simulink model "MaIA_SDCI_Temperature_Control"  (R2025b)
settings: Solver=VariableStepAuto  StartTime=0.0  StopTime=1800  RelTol=1e-3
PreLoadFcn:
  | %% MaIA_SDCI - Model Preload Callback
  | % Keep this callback intentionally minimal.
  | % All portable initialization logic lives in startup_project.m.
  | 
  | modelFile = get_param(bdroot, 'FileName');
  | 
  | if isempty(modelFile)
  |     error('MaIA_SDCI:ModelFileNotFound', ...
  |         'Unable to determine the current model file location.');
  | end
  | 
  | projectRoot = fileparts(modelFile);
  | addpath(projectRoot, '-begin');
  | rehash path;
  | startup_project(projectRoot);
InitFcn:
  | %% ============================================================
  | %  SIMULATION LAUNCH SOURCE
  | %  ============================================================
  | 
  | % false -> Run initiated directly from Simulink
  | % true  -> Run initiated from the MaIA_SDCI GUI
  | %
  | % Do not overwrite this variable if it already exists because
  | % the GUI sets it to true immediately before starting a run.
  | 
  | if ~evalin( ...
  |         'base', ...
  |         'exist(''MaIA_SDCI_RUN_FROM_GUI'',''var'')')
  | 
  |     assignin( ...
  |         'base', ...
  |         'MaIA_SDCI_RUN_FROM_GUI', ...
  |         false);
  | 
  | end
StartFcn:
  | %% MaIA_SDCI - Simulation Start Callback
  | 
  | runFromGUI = false;
  | 
  | %% Check simulation origin
  | 
  | if evalin( ...
  |         'base', ...
  |         'exist(''MaIA_SDCI_RUN_FROM_GUI'',''var'')')
  | 
  |     flagValue = evalin( ...
  |         'base', ...
  |         'MaIA_SDCI_RUN_FROM_GUI');
  | 
  |     if islogical(flagValue) || isnumeric(flagValue)
  |         runFromGUI = logical(flagValue);
  |     end
  | 
  | end
  | 
  | %% Open or focus the control application
  | 
  | launch_app;
  | 
  | %% Manual Run from Simulink
  | 
  | if ~runFromGUI
  | 
  |     drawnow;
  | 
  |     set_param( ...
  |         bdroot, ...
  |         'SimulationCommand', ...
  |         'stop');
  | 
  | end
values from neighbouring files (symbols this model uses):
  CFG = project_config()    [startup_project.m]
  ENV = environment_parameters()    [startup_project.m]
  MODEL = model_parameters()    [startup_project.m]
  SENSOR = sensor_parameters()    [startup_project.m]
libraries: fl_lib x58, nesl_utility x38, simulink x2
(part 2 of 2)

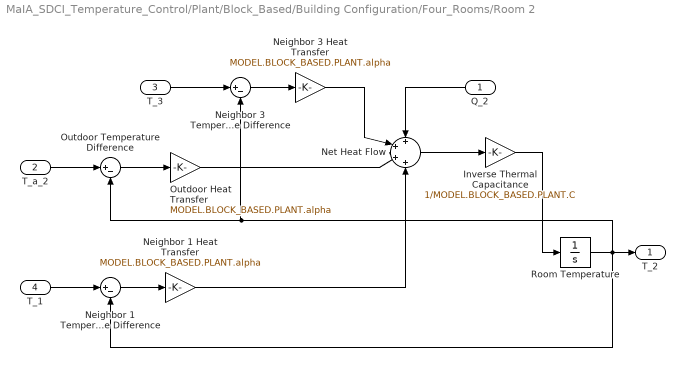
== system MaIA_SDCI_Temperature_Control/Plant/Block_Based/Building Configuration/Four_Rooms/Room 2 ==
  Q_2 : Inport
  T_a_2 : Inport  Port=2
  T_3 : Inport  Port=3
  T_1 : Inport  Port=4
  Inverse Thermal Capacitance : Gain  Gain=1/MODEL.BLOCK_BASED.PLANT.C
  Neighbor 1 Heat Transfer : Gain  Gain=MODEL.BLOCK_BASED.PLANT.alpha
  Neighbor 1 Temperature Difference : Sum  Inputs=|+-
  Neighbor 3 Heat Transfer : Gain  Gain=MODEL.BLOCK_BASED.PLANT.alpha
  Neighbor 3 Temperature Difference : Sum  Inputs=|+-
  Net Heat Flow : Sum  Inputs=++++
  Outdoor Heat Transfer : Gain  Gain=MODEL.BLOCK_BASED.PLANT.alpha
  Outdoor Temperature Difference : Sum  Inputs=|+-
  Room Temperature : Integrator  InitialCondition=MODEL.BLOCK_BASED.PLANT.initialTemperature(2)
  T_2 : Outport
  wires:
  Room Temperature/1 -> Neighbor 3 Temperature Difference/2, Outdoor Temperature Difference/2, T_2/1, Neighbor 1 Temperature Difference/2
  T_a_2/1 -> Outdoor Temperature Difference/1
  Outdoor Temperature Difference/1 -> Outdoor Heat Transfer/1
  T_1/1 -> Neighbor 1 Temperature Difference/1
  Neighbor 1 Temperature Difference/1 -> Neighbor 1 Heat Transfer/1
  T_3/1 -> Neighbor 3 Temperature Difference/1
  Neighbor 3 Temperature Difference/1 -> Neighbor 3 Heat Transfer/1
  Neighbor 3 Heat Transfer/1 -> Net Heat Flow/2
  Q_2/1 -> Net Heat Flow/1
  Neighbor 1 Heat Transfer/1 -> Net Heat Flow/4
  Outdoor Heat Transfer/1 -> Net Heat Flow/3
  Net Heat Flow/1 -> Inverse Thermal Capacitance/1
  Inverse Thermal Capacitance/1 -> Room Temperature/1

== system MaIA_SDCI_Temperature_Control/Plant/Block_Based/Building Configuration/Four_Rooms/Room 3 ==
  Q_3 : Inport
  T_a_3 : Inport  Port=2
  T_4 : Inport  Port=3
  T_2 : Inport  Port=4
  Inverse Thermal Capacitance : Gain  Gain=1/MODEL.BLOCK_BASED.PLANT.C
  Neighbor 2 Heat Transfer : Gain  Gain=MODEL.BLOCK_BASED.PLANT.alpha
  Neighbor 2 Temperature Difference : Sum  Inputs=|+-
  Neighbor 4 Heat Transfer : Gain  Gain=MODEL.BLOCK_BASED.PLANT.alpha
  Neighbor 4 Temperature Difference : Sum  Inputs=|+-
  Net Heat Flow : Sum  Inputs=++++
  Outdoor Heat Transfer : Gain  Gain=MODEL.BLOCK_BASED.PLANT.alpha
  Outdoor Temperature Difference : Sum  Inputs=|+-
  Room Temperature : Integrator  InitialCondition=MODEL.BLOCK_BASED.PLANT.initialTemperature(3)
  T_3 : Outport
  wires:
  Room Temperature/1 -> Neighbor 4 Temperature Difference/2, Outdoor Temperature Difference/2, T_3/1, Neighbor 2 Temperature Difference/2
  T_a_3/1 -> Outdoor Temperature Difference/1
  Outdoor Temperature Difference/1 -> Outdoor Heat Transfer/1
  T_2/1 -> Neighbor 2 Temperature Difference/1
  Neighbor 2 Temperature Difference/1 -> Neighbor 2 Heat Transfer/1
  T_4/1 -> Neighbor 4 Temperature Difference/1
  Neighbor 4 Temperature Difference/1 -> Neighbor 4 Heat Transfer/1
  Neighbor 4 Heat Transfer/1 -> Net Heat Flow/2
  Q_3/1 -> Net Heat Flow/1
  Neighbor 2 Heat Transfer/1 -> Net Heat Flow/4
  Outdoor Heat Transfer/1 -> Net Heat Flow/3
  Net Heat Flow/1 -> Inverse Thermal Capacitance/1
  Inverse Thermal Capacitance/1 -> Room Temperature/1

== system MaIA_SDCI_Temperature_Control/Plant/Block_Based/Building Configuration/Four_Rooms/Room 4 ==
  Q_4 : Inport
  T_a_4 : Inport  Port=2
  T_3 : Inport  Port=3
  Inverse Thermal Capacitance : Gain  Gain=1/MODEL.BLOCK_BASED.PLANT.C
  Neighbor 3 Heat Transfer : Gain  Gain=MODEL.BLOCK_BASED.PLANT.alpha
  Neighbor 3 Temperature Difference : Sum  Inputs=|+-
  Net Heat Flow : Sum  Inputs=|+++
  Outdoor Heat Transfer : Gain  Gain=MODEL.BLOCK_BASED.PLANT.alpha
  Outdoor Temperature Difference : Sum  Inputs=|+-
  Room Temperature : Integrator  InitialCondition=MODEL.BLOCK_BASED.PLANT.initialTemperature(4)
  T_4 : Outport
  wires:
  T_a_4/1 -> Outdoor Temperature Difference/1
  Room Temperature/1 -> Neighbor 3 Temperature Difference/2, T_4/1, Outdoor Temperature Difference/2
  Outdoor Temperature Difference/1 -> Outdoor Heat Transfer/1
  T_3/1 -> Neighbor 3 Temperature Difference/1
  Neighbor 3 Temperature Difference/1 -> Neighbor 3 Heat Transfer/1
  Outdoor Heat Transfer/1 -> Net Heat Flow/2
  Neighbor 3 Heat Transfer/1 -> Net Heat Flow/3
  Q_4/1 -> Net Heat Flow/1
  Net Heat Flow/1 -> Inverse Thermal Capacitance/1
  Inverse Thermal Capacitance/1 -> Room Temperature/1

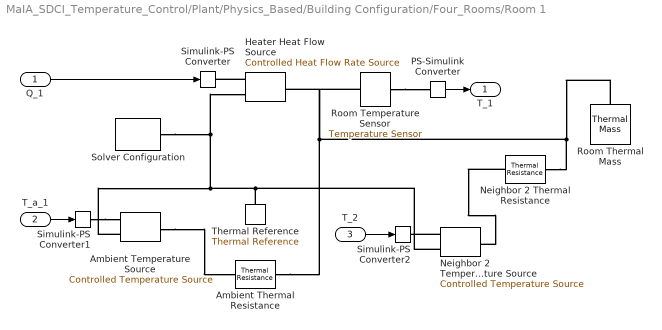
== system MaIA_SDCI_Temperature_Control/Plant/Physics_Based/Building Configuration/Four_Rooms/Room 1 ==
  Q_1 : Inport
  T_a_1 : Inport  Port=2
  T_2 : Inport  Port=3
  " Thermal Reference" : fl_lib/Thermal/Thermal Elements/Thermal Reference
  Ambient Temperature Source : fl_lib/Thermal/Thermal Sources/Controlled Temperature Source
  Ambient Thermal Resistance : fl_lib/Thermal/Thermal Elements/Thermal Resistance  resistance=1/MODEL.SIMSCAPE.PLANT.alpha K/W  T_specify=off  T_priority=None  T=0 K  T_nominal_specify=off  T_nominal_value=1  T_nominal_unit=K  Q_specify=off  Q_priority=None  Q=0 W  Q_nominal_specify=off  Q_nominal_value=1  Q_nominal_unit=W
  "Heater Heat Flow Source " : fl_lib/Thermal/Thermal Sources/Controlled Heat Flow Rate Source
  Neighbor 2 Temperature Source : fl_lib/Thermal/Thermal Sources/Controlled Temperature Source
  Neighbor 2 Thermal Resistance : fl_lib/Thermal/Thermal Elements/Thermal Resistance  resistance=1/MODEL.SIMSCAPE.PLANT.alpha K/W  T_specify=off  T_priority=None  T=0 K  T_nominal_specify=off  T_nominal_value=1  T_nominal_unit=K  Q_specify=off  Q_priority=None  Q=0 W  Q_nominal_specify=off  Q_nominal_value=1  Q_nominal_unit=W
  PS-Simulink Converter : nesl_utility/PS-Simulink Converter  PhysicalDomain=network_engine_domain  SubClassName=ps_output  LeftPortType=input  RightPortType=output  PseudoPeriodic=off  Frequencies=[]  VectorFormat=inherit  Unit=degC  AffineConversion=on
  Room Temperature Sensor : fl_lib/Thermal/Thermal Sensors/Temperature Sensor  temperature_measure=foundation.enum.MeasurementReference.absolute
      settings: InternalSimscapePortConfiguration="{\"Bottom\":[],\"Left\":[{\"id\":\"A\",\"label\":\"A\",\"type\":\"foundation.thermal.thermal\"}],\"Right\":[{\"id\":\"T\",\"label\":\"T\",\"type\":\"output\"}],\"Top\":[]}"
  Room Thermal Mass : fl_lib/Thermal/Thermal Elements/Thermal Mass  mass_type=foundation.enum.constant_variable.constant  mass=1 kg  sp_heat=MODEL.SIMSCAPE.PLANT.C J/(K*kg)  mass_min=1e-6 kg  num_ports=foundation.enum.numPorts2.one  m_specify=off  m_priority=High  m=1 kg  m_nominal_specify=off  m_nominal_value=1  m_nominal_unit=kg  T_specify=on  T_priority=High  T=MODEL.SIMSCAPE.PLANT.initialTemperature(1) degC  T_nominal_specify=off  T_nominal_value=1  T_nominal_unit=K  Q_specify=off  Q_priority=None  Q=0 W  Q_nominal_specify=off  Q_nominal_value=1  Q_nominal_unit=W
  Simulink-PS Converter : nesl_utility/Simulink-PS Converter  PhysicalDomain=network_engine_domain  SubClassName=ps_input  LeftPortType=input  RightPortType=output  PseudoPeriodic=off  Frequencies=[]  NoiseDistribution=none  NoiseParameters=[]  Unit=W  AffineConversion=off  FilteringAndDerivatives=provide  SimscapeFilterOrder=1  InputFilterTimeConstant=0.001  UdotUserProvided=0
  Simulink-PS Converter1 : nesl_utility/Simulink-PS Converter  PhysicalDomain=network_engine_domain  SubClassName=ps_input  LeftPortType=input  RightPortType=output  PseudoPeriodic=off  Frequencies=[]  NoiseDistribution=none  NoiseParameters=[]  Unit=degC  AffineConversion=on  FilteringAndDerivatives=provide  SimscapeFilterOrder=1  InputFilterTimeConstant=0.001  UdotUserProvided=0
  Simulink-PS Converter2 : nesl_utility/Simulink-PS Converter  PhysicalDomain=network_engine_domain  SubClassName=ps_input  LeftPortType=input  RightPortType=output  PseudoPeriodic=off  Frequencies=[]  NoiseDistribution=none  NoiseParameters=[]  Unit=degC  AffineConversion=on  FilteringAndDerivatives=provide  SimscapeFilterOrder=1  InputFilterTimeConstant=0.001  UdotUserProvided=0
  "Solver Configuration " : nesl_utility/Solver Configuration  PhysicalDomain=network_engine_domain  SubClassName=solver  LeftPortType=input  RightPortType=generic  Tones=[]  Harmonics=[]  SimulateNoise=off  Profile=off  UseLocalSampling=off  EnableSwitchedLinearOptims=on  FrequencyDomain=off  UseCCode=off  RelTol=0.001  AbsTol=0.001  MinStep=1e-09  ToWorkspace=off  RevertToSquareIcSolve=off  NumHomotopyIterations=100  PhasorMode=off  PhasorModeNumHarmonics=1  ConsistencySolver=NEWTON_XTOL_AFTER_FTOL  IndexReductionMethod=DerivativeReplacement  DoDC=off  ResidualTolerance=1e-09  ConsistencyTolSource=GLOBAL  ConsistencyAbsTol=0.001  ConsistencyRelTol=0.001  ConsistencyTolFactor=0.001  UseLocalSolver=off  LocalSolverChoice=NE_BACKWARD_EULER_ADVANCER  ResolveIndetEquations=on  FunctionEvalNumThread=1  LocalSolverSampleTime=0.001  DoFixedCost=off  MaxNonlinIter=3  MaxModeIter=2  ComputeImpulses=off  ImpulseIterations=2  LinearAlgebra=auto  LinearAlgebraNumThread=0  EquationFormulation=NE_TIME_EF  DelaysMemoryBudget=1024  AutomaticFiltering=on  FilteringTimeConstant=0.001  PartitionStorageMethod=AS_NEEDED  PartitionMemoryBudget=1024  PartitionMethod=ROBUST  MultibodyUseLocalSolver=off  MultibodyLocalSolverChoice=ODE1  MultibodyLocalSolverSampleTime=0.001
  T_1 : Outport
  wires:
  Q_1/1 -> Simulink-PS Converter/1
  PS-Simulink Converter/1 -> T_1/1
  T_a_1/1 -> Simulink-PS Converter1/1
  T_2/1 -> Simulink-PS Converter2/1
  connections:
  "Heater Heat Flow Source "/RConn1 -- Simulink-PS Converter/RConn1
  Room Thermal Mass/LConn1 -- Room Temperature Sensor/LConn1 -- "Heater Heat Flow Source "/LConn1 -- Ambient Thermal Resistance/RConn1 -- Neighbor 2 Thermal Resistance/RConn1
  Room Temperature Sensor/RConn1 -- PS-Simulink Converter/LConn1
  " Thermal Reference"/LConn1 -- Neighbor 2 Temperature Source/RConn2 -- "Solver Configuration "/RConn1 -- "Heater Heat Flow Source "/RConn2 -- Ambient Temperature Source/RConn2
  Simulink-PS Converter1/RConn1 -- Ambient Temperature Source/RConn1
  Neighbor 2 Temperature Source/RConn1 -- Simulink-PS Converter2/RConn1
  Ambient Temperature Source/LConn1 -- Ambient Thermal Resistance/LConn1
  Neighbor 2 Thermal Resistance/LConn1 -- Neighbor 2 Temperature Source/LConn1

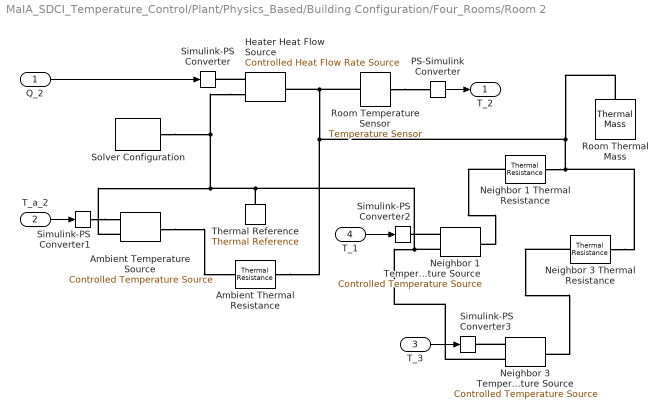
== system MaIA_SDCI_Temperature_Control/Plant/Physics_Based/Building Configuration/Four_Rooms/Room 2 ==
  Q_2 : Inport
  T_a_2 : Inport  Port=2
  T_3 : Inport  Port=3
  T_1 : Inport  Port=4
  " Thermal Reference" : fl_lib/Thermal/Thermal Elements/Thermal Reference
  Ambient Temperature Source : fl_lib/Thermal/Thermal Sources/Controlled Temperature Source
  Ambient Thermal Resistance : fl_lib/Thermal/Thermal Elements/Thermal Resistance  resistance=1/MODEL.SIMSCAPE.PLANT.alpha K/W  T_specify=off  T_priority=None  T=0 K  T_nominal_specify=off  T_nominal_value=1  T_nominal_unit=K  Q_specify=off  Q_priority=None  Q=0 W  Q_nominal_specify=off  Q_nominal_value=1  Q_nominal_unit=W
  "Heater Heat Flow Source " : fl_lib/Thermal/Thermal Sources/Controlled Heat Flow Rate Source
  Neighbor 1 Temperature Source : fl_lib/Thermal/Thermal Sources/Controlled Temperature Source
  Neighbor 1 Thermal Resistance : fl_lib/Thermal/Thermal Elements/Thermal Resistance  resistance=1/MODEL.SIMSCAPE.PLANT.alpha K/W  T_specify=off  T_priority=None  T=0 K  T_nominal_specify=off  T_nominal_value=1  T_nominal_unit=K  Q_specify=off  Q_priority=None  Q=0 W  Q_nominal_specify=off  Q_nominal_value=1  Q_nominal_unit=W
  Neighbor 3 Temperature Source : fl_lib/Thermal/Thermal Sources/Controlled Temperature Source
  Neighbor 3 Thermal Resistance : fl_lib/Thermal/Thermal Elements/Thermal Resistance  resistance=1/MODEL.SIMSCAPE.PLANT.alpha K/W  T_specify=off  T_priority=None  T=0 K  T_nominal_specify=off  T_nominal_value=1  T_nominal_unit=K  Q_specify=off  Q_priority=None  Q=0 W  Q_nominal_specify=off  Q_nominal_value=1  Q_nominal_unit=W
  PS-Simulink Converter : nesl_utility/PS-Simulink Converter  PhysicalDomain=network_engine_domain  SubClassName=ps_output  LeftPortType=input  RightPortType=output  PseudoPeriodic=off  Frequencies=[]  VectorFormat=inherit  Unit=degC  AffineConversion=on
  Room Temperature Sensor : fl_lib/Thermal/Thermal Sensors/Temperature Sensor  temperature_measure=foundation.enum.MeasurementReference.absolute
      settings: InternalSimscapePortConfiguration="{\"Bottom\":[],\"Left\":[{\"id\":\"A\",\"label\":\"A\",\"type\":\"foundation.thermal.thermal\"}],\"Right\":[{\"id\":\"T\",\"label\":\"T\",\"type\":\"output\"}],\"Top\":[]}"
  Room Thermal Mass : fl_lib/Thermal/Thermal Elements/Thermal Mass  mass_type=foundation.enum.constant_variable.constant  mass=1 kg  sp_heat=MODEL.SIMSCAPE.PLANT.C J/(K*kg)  mass_min=1e-6 kg  num_ports=foundation.enum.numPorts2.one  m_specify=off  m_priority=High  m=1 kg  m_nominal_specify=off  m_nominal_value=1  m_nominal_unit=kg  T_specify=on  T_priority=High  T=MODEL.SIMSCAPE.PLANT.initialTemperature(2) degC  T_nominal_specify=off  T_nominal_value=1  T_nominal_unit=K  Q_specify=off  Q_priority=None  Q=0 W  Q_nominal_specify=off  Q_nominal_value=1  Q_nominal_unit=W
  Simulink-PS Converter : nesl_utility/Simulink-PS Converter  PhysicalDomain=network_engine_domain  SubClassName=ps_input  LeftPortType=input  RightPortType=output  PseudoPeriodic=off  Frequencies=[]  NoiseDistribution=none  NoiseParameters=[]  Unit=W  AffineConversion=off  FilteringAndDerivatives=provide  SimscapeFilterOrder=1  InputFilterTimeConstant=0.001  UdotUserProvided=0
  Simulink-PS Converter1 : nesl_utility/Simulink-PS Converter  PhysicalDomain=network_engine_domain  SubClassName=ps_input  LeftPortType=input  RightPortType=output  PseudoPeriodic=off  Frequencies=[]  NoiseDistribution=none  NoiseParameters=[]  Unit=degC  AffineConversion=on  FilteringAndDerivatives=provide  SimscapeFilterOrder=1  InputFilterTimeConstant=0.001  UdotUserProvided=0
  Simulink-PS Converter2 : nesl_utility/Simulink-PS Converter  PhysicalDomain=network_engine_domain  SubClassName=ps_input  LeftPortType=input  RightPortType=output  PseudoPeriodic=off  Frequencies=[]  NoiseDistribution=none  NoiseParameters=[]  Unit=degC  AffineConversion=on  FilteringAndDerivatives=provide  SimscapeFilterOrder=1  InputFilterTimeConstant=0.001  UdotUserProvided=0
  Simulink-PS Converter3 : nesl_utility/Simulink-PS Converter  PhysicalDomain=network_engine_domain  SubClassName=ps_input  LeftPortType=input  RightPortType=output  PseudoPeriodic=off  Frequencies=[]  NoiseDistribution=none  NoiseParameters=[]  Unit=degC  AffineConversion=on  FilteringAndDerivatives=provide  SimscapeFilterOrder=1  InputFilterTimeConstant=0.001  UdotUserProvided=0
  "Solver Configuration " : nesl_utility/Solver Configuration  PhysicalDomain=network_engine_domain  SubClassName=solver  LeftPortType=input  RightPortType=generic  Tones=[]  Harmonics=[]  SimulateNoise=off  Profile=off  UseLocalSampling=off  EnableSwitchedLinearOptims=on  FrequencyDomain=off  UseCCode=off  RelTol=0.001  AbsTol=0.001  MinStep=1e-09  ToWorkspace=off  RevertToSquareIcSolve=off  NumHomotopyIterations=100  PhasorMode=off  PhasorModeNumHarmonics=1  ConsistencySolver=NEWTON_XTOL_AFTER_FTOL  IndexReductionMethod=DerivativeReplacement  DoDC=off  ResidualTolerance=1e-09  ConsistencyTolSource=GLOBAL  ConsistencyAbsTol=0.001  ConsistencyRelTol=0.001  ConsistencyTolFactor=0.001  UseLocalSolver=off  LocalSolverChoice=NE_BACKWARD_EULER_ADVANCER  ResolveIndetEquations=on  FunctionEvalNumThread=1  LocalSolverSampleTime=0.001  DoFixedCost=off  MaxNonlinIter=3  MaxModeIter=2  ComputeImpulses=off  ImpulseIterations=2  LinearAlgebra=auto  LinearAlgebraNumThread=0  EquationFormulation=NE_TIME_EF  DelaysMemoryBudget=1024  AutomaticFiltering=on  FilteringTimeConstant=0.001  PartitionStorageMethod=AS_NEEDED  PartitionMemoryBudget=1024  PartitionMethod=ROBUST  MultibodyUseLocalSolver=off  MultibodyLocalSolverChoice=ODE1  MultibodyLocalSolverSampleTime=0.001
  T_2 : Outport
  wires:
  T_1/1 -> Simulink-PS Converter2/1
  T_a_2/1 -> Simulink-PS Converter1/1
  PS-Simulink Converter/1 -> T_2/1
  Q_2/1 -> Simulink-PS Converter/1
  T_3/1 -> Simulink-PS Converter3/1
  connections:
  "Heater Heat Flow Source "/RConn2 -- " Thermal Reference"/LConn1 -- Neighbor 3 Temperature Source/RConn2 -- Neighbor 1 Temperature Source/RConn2 -- Ambient Temperature Source/RConn2 -- "Solver Configuration "/RConn1
  Room Thermal Mass/LConn1 -- Room Temperature Sensor/LConn1 -- "Heater Heat Flow Source "/LConn1 -- Ambient Thermal Resistance/RConn1 -- Neighbor 1 Thermal Resistance/RConn1 -- Neighbor 3 Thermal Resistance/RConn1
  Neighbor 1 Thermal Resistance/LConn1 -- Neighbor 1 Temperature Source/LConn1
  Room Temperature Sensor/RConn1 -- PS-Simulink Converter/LConn1
  Simulink-PS Converter1/RConn1 -- Ambient Temperature Source/RConn1
  Neighbor 1 Temperature Source/RConn1 -- Simulink-PS Converter2/RConn1
  "Heater Heat Flow Source "/RConn1 -- Simulink-PS Converter/RConn1
  Ambient Temperature Source/LConn1 -- Ambient Thermal Resistance/LConn1
  Neighbor 3 Temperature Source/RConn1 -- Simulink-PS Converter3/RConn1
  Neighbor 3 Thermal Resistance/LConn1 -- Neighbor 3 Temperature Source/LConn1

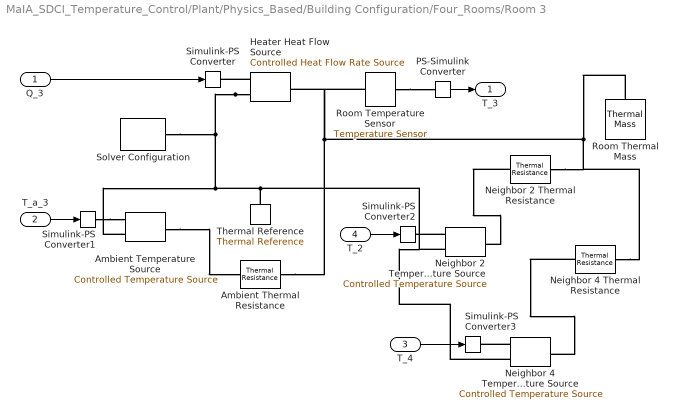
== system MaIA_SDCI_Temperature_Control/Plant/Physics_Based/Building Configuration/Four_Rooms/Room 3 ==
  Q_3 : Inport
  T_a_3 : Inport  Port=2
  T_4 : Inport  Port=3
  T_2 : Inport  Port=4
  " Thermal Reference" : fl_lib/Thermal/Thermal Elements/Thermal Reference
  Ambient Temperature Source : fl_lib/Thermal/Thermal Sources/Controlled Temperature Source
  Ambient Thermal Resistance : fl_lib/Thermal/Thermal Elements/Thermal Resistance  resistance=1/MODEL.SIMSCAPE.PLANT.alpha K/W  T_specify=off  T_priority=None  T=0 K  T_nominal_specify=off  T_nominal_value=1  T_nominal_unit=K  Q_specify=off  Q_priority=None  Q=0 W  Q_nominal_specify=off  Q_nominal_value=1  Q_nominal_unit=W
  Heater Heat Flow Source : fl_lib/Thermal/Thermal Sources/Controlled Heat Flow Rate Source
  Neighbor 2 Temperature Source : fl_lib/Thermal/Thermal Sources/Controlled Temperature Source
  Neighbor 2 Thermal Resistance : fl_lib/Thermal/Thermal Elements/Thermal Resistance  resistance=1/MODEL.SIMSCAPE.PLANT.alpha K/W  T_specify=off  T_priority=None  T=0 K  T_nominal_specify=off  T_nominal_value=1  T_nominal_unit=K  Q_specify=off  Q_priority=None  Q=0 W  Q_nominal_specify=off  Q_nominal_value=1  Q_nominal_unit=W
  Neighbor 4 Temperature Source : fl_lib/Thermal/Thermal Sources/Controlled Temperature Source
  Neighbor 4 Thermal Resistance : fl_lib/Thermal/Thermal Elements/Thermal Resistance  resistance=1/MODEL.SIMSCAPE.PLANT.alpha K/W  T_specify=off  T_priority=None  T=0 K  T_nominal_specify=off  T_nominal_value=1  T_nominal_unit=K  Q_specify=off  Q_priority=None  Q=0 W  Q_nominal_specify=off  Q_nominal_value=1  Q_nominal_unit=W
  PS-Simulink Converter : nesl_utility/PS-Simulink Converter  PhysicalDomain=network_engine_domain  SubClassName=ps_output  LeftPortType=input  RightPortType=output  PseudoPeriodic=off  Frequencies=[]  VectorFormat=inherit  Unit=degC  AffineConversion=on
  Room Temperature Sensor : fl_lib/Thermal/Thermal Sensors/Temperature Sensor  temperature_measure=foundation.enum.MeasurementReference.absolute
      settings: InternalSimscapePortConfiguration="{\"Bottom\":[],\"Left\":[{\"id\":\"A\",\"label\":\"A\",\"type\":\"foundation.thermal.thermal\"}],\"Right\":[{\"id\":\"T\",\"label\":\"T\",\"type\":\"output\"}],\"Top\":[]}"
  Room Thermal Mass : fl_lib/Thermal/Thermal Elements/Thermal Mass  mass_type=foundation.enum.constant_variable.constant  mass=1 kg  sp_heat=MODEL.SIMSCAPE.PLANT.C J/(K*kg)  mass_min=1e-6 kg  num_ports=foundation.enum.numPorts2.one  m_specify=off  m_priority=High  m=1 kg  m_nominal_specify=off  m_nominal_value=1  m_nominal_unit=kg  T_specify=on  T_priority=High  T=MODEL.SIMSCAPE.PLANT.initialTemperature(3) degC  T_nominal_specify=off  T_nominal_value=1  T_nominal_unit=K  Q_specify=off  Q_priority=None  Q=0 W  Q_nominal_specify=off  Q_nominal_value=1  Q_nominal_unit=W
  Simulink-PS Converter : nesl_utility/Simulink-PS Converter  PhysicalDomain=network_engine_domain  SubClassName=ps_input  LeftPortType=input  RightPortType=output  PseudoPeriodic=off  Frequencies=[]  NoiseDistribution=none  NoiseParameters=[]  Unit=W  AffineConversion=off  FilteringAndDerivatives=provide  SimscapeFilterOrder=1  InputFilterTimeConstant=0.001  UdotUserProvided=0
  Simulink-PS Converter1 : nesl_utility/Simulink-PS Converter  PhysicalDomain=network_engine_domain  SubClassName=ps_input  LeftPortType=input  RightPortType=output  PseudoPeriodic=off  Frequencies=[]  NoiseDistribution=none  NoiseParameters=[]  Unit=degC  AffineConversion=on  FilteringAndDerivatives=provide  SimscapeFilterOrder=1  InputFilterTimeConstant=0.001  UdotUserProvided=0
  Simulink-PS Converter2 : nesl_utility/Simulink-PS Converter  PhysicalDomain=network_engine_domain  SubClassName=ps_input  LeftPortType=input  RightPortType=output  PseudoPeriodic=off  Frequencies=[]  NoiseDistribution=none  NoiseParameters=[]  Unit=degC  AffineConversion=on  FilteringAndDerivatives=provide  SimscapeFilterOrder=1  InputFilterTimeConstant=0.001  UdotUserProvided=0
  Simulink-PS Converter3 : nesl_utility/Simulink-PS Converter  PhysicalDomain=network_engine_domain  SubClassName=ps_input  LeftPortType=input  RightPortType=output  PseudoPeriodic=off  Frequencies=[]  NoiseDistribution=none  NoiseParameters=[]  Unit=degC  AffineConversion=on  FilteringAndDerivatives=provide  SimscapeFilterOrder=1  InputFilterTimeConstant=0.001  UdotUserProvided=0
  "Solver Configuration " : nesl_utility/Solver Configuration  PhysicalDomain=network_engine_domain  SubClassName=solver  LeftPortType=input  RightPortType=generic  Tones=[]  Harmonics=[]  SimulateNoise=off  Profile=off  UseLocalSampling=off  EnableSwitchedLinearOptims=on  FrequencyDomain=off  UseCCode=off  RelTol=0.001  AbsTol=0.001  MinStep=1e-09  ToWorkspace=off  RevertToSquareIcSolve=off  NumHomotopyIterations=100  PhasorMode=off  PhasorModeNumHarmonics=1  ConsistencySolver=NEWTON_XTOL_AFTER_FTOL  IndexReductionMethod=DerivativeReplacement  DoDC=off  ResidualTolerance=1e-09  ConsistencyTolSource=GLOBAL  ConsistencyAbsTol=0.001  ConsistencyRelTol=0.001  ConsistencyTolFactor=0.001  UseLocalSolver=off  LocalSolverChoice=NE_BACKWARD_EULER_ADVANCER  ResolveIndetEquations=on  FunctionEvalNumThread=1  LocalSolverSampleTime=0.001  DoFixedCost=off  MaxNonlinIter=3  MaxModeIter=2  ComputeImpulses=off  ImpulseIterations=2  LinearAlgebra=auto  LinearAlgebraNumThread=0  EquationFormulation=NE_TIME_EF  DelaysMemoryBudget=1024  AutomaticFiltering=on  FilteringTimeConstant=0.001  PartitionStorageMethod=AS_NEEDED  PartitionMemoryBudget=1024  PartitionMethod=ROBUST  MultibodyUseLocalSolver=off  MultibodyLocalSolverChoice=ODE1  MultibodyLocalSolverSampleTime=0.001
  T_3 : Outport
  wires:
  T_a_3/1 -> Simulink-PS Converter1/1
  PS-Simulink Converter/1 -> T_3/1
  Q_3/1 -> Simulink-PS Converter/1
  T_2/1 -> Simulink-PS Converter2/1
  T_4/1 -> Simulink-PS Converter3/1
  connections:
  Room Thermal Mass/LConn1 -- Room Temperature Sensor/LConn1 -- Heater Heat Flow Source/LConn1 -- Ambient Thermal Resistance/RConn1 -- Neighbor 2 Thermal Resistance/RConn1 -- Neighbor 4 Thermal Resistance/RConn1
  Heater Heat Flow Source/RConn2 -- "Solver Configuration "/RConn1 -- Ambient Temperature Source/RConn2 -- " Thermal Reference"/LConn1 -- Neighbor 4 Temperature Source/RConn2 -- Neighbor 2 Temperature Source/RConn2
  Heater Heat Flow Source/RConn1 -- Simulink-PS Converter/RConn1
  Neighbor 2 Temperature Source/RConn1 -- Simulink-PS Converter2/RConn1
  Neighbor 2 Thermal Resistance/LConn1 -- Neighbor 2 Temperature Source/LConn1
  Ambient Temperature Source/LConn1 -- Ambient Thermal Resistance/LConn1
  Neighbor 4 Thermal Resistance/LConn1 -- Neighbor 4 Temperature Source/LConn1
  Neighbor 4 Temperature Source/RConn1 -- Simulink-PS Converter3/RConn1
  Room Temperature Sensor/RConn1 -- PS-Simulink Converter/LConn1
  Simulink-PS Converter1/RConn1 -- Ambient Temperature Source/RConn1

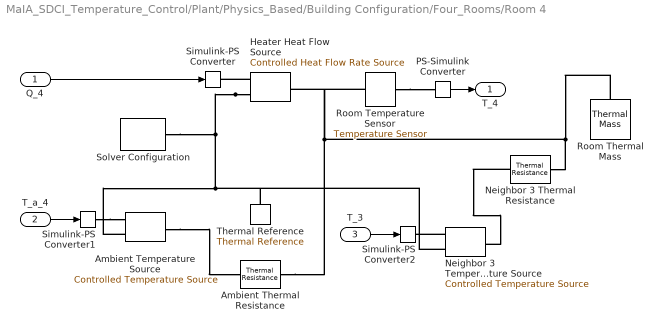
== system MaIA_SDCI_Temperature_Control/Plant/Physics_Based/Building Configuration/Four_Rooms/Room 4 ==
  Q_4 : Inport
  T_a_4 : Inport  Port=2
  T_3 : Inport  Port=3
  " Thermal Reference" : fl_lib/Thermal/Thermal Elements/Thermal Reference
  Ambient Temperature Source : fl_lib/Thermal/Thermal Sources/Controlled Temperature Source
  Ambient Thermal Resistance : fl_lib/Thermal/Thermal Elements/Thermal Resistance  resistance=1/MODEL.SIMSCAPE.PLANT.alpha K/W  T_specify=off  T_priority=None  T=0 K  T_nominal_specify=off  T_nominal_value=1  T_nominal_unit=K  Q_specify=off  Q_priority=None  Q=0 W  Q_nominal_specify=off  Q_nominal_value=1  Q_nominal_unit=W
  "Heater Heat Flow Source " : fl_lib/Thermal/Thermal Sources/Controlled Heat Flow Rate Source
  Neighbor 3 Temperature Source : fl_lib/Thermal/Thermal Sources/Controlled Temperature Source
  Neighbor 3 Thermal Resistance : fl_lib/Thermal/Thermal Elements/Thermal Resistance  resistance=1/MODEL.SIMSCAPE.PLANT.alpha K/W  T_specify=off  T_priority=None  T=0 K  T_nominal_specify=off  T_nominal_value=1  T_nominal_unit=K  Q_specify=off  Q_priority=None  Q=0 W  Q_nominal_specify=off  Q_nominal_value=1  Q_nominal_unit=W
  PS-Simulink Converter : nesl_utility/PS-Simulink Converter  PhysicalDomain=network_engine_domain  SubClassName=ps_output  LeftPortType=input  RightPortType=output  PseudoPeriodic=off  Frequencies=[]  VectorFormat=inherit  Unit=degC  AffineConversion=on
  Room Temperature Sensor : fl_lib/Thermal/Thermal Sensors/Temperature Sensor  temperature_measure=foundation.enum.MeasurementReference.absolute
      settings: InternalSimscapePortConfiguration="{\"Bottom\":[],\"Left\":[{\"id\":\"A\",\"label\":\"A\",\"type\":\"foundation.thermal.thermal\"}],\"Right\":[{\"id\":\"T\",\"label\":\"T\",\"type\":\"output\"}],\"Top\":[]}"
  Room Thermal Mass : fl_lib/Thermal/Thermal Elements/Thermal Mass  mass_type=foundation.enum.constant_variable.constant  mass=1 kg  sp_heat=MODEL.SIMSCAPE.PLANT.C J/(K*kg)  mass_min=1e-6 kg  num_ports=foundation.enum.numPorts2.one  m_specify=off  m_priority=High  m=1 kg  m_nominal_specify=off  m_nominal_value=1  m_nominal_unit=kg  T_specify=on  T_priority=High  T=MODEL.SIMSCAPE.PLANT.initialTemperature(4) degC  T_nominal_specify=off  T_nominal_value=1  T_nominal_unit=K  Q_specify=off  Q_priority=None  Q=0 W  Q_nominal_specify=off  Q_nominal_value=1  Q_nominal_unit=W
  Simulink-PS Converter : nesl_utility/Simulink-PS Converter  PhysicalDomain=network_engine_domain  SubClassName=ps_input  LeftPortType=input  RightPortType=output  PseudoPeriodic=off  Frequencies=[]  NoiseDistribution=none  NoiseParameters=[]  Unit=W  AffineConversion=off  FilteringAndDerivatives=provide  SimscapeFilterOrder=1  InputFilterTimeConstant=0.001  UdotUserProvided=0
  Simulink-PS Converter1 : nesl_utility/Simulink-PS Converter  PhysicalDomain=network_engine_domain  SubClassName=ps_input  LeftPortType=input  RightPortType=output  PseudoPeriodic=off  Frequencies=[]  NoiseDistribution=none  NoiseParameters=[]  Unit=degC  AffineConversion=on  FilteringAndDerivatives=provide  SimscapeFilterOrder=1  InputFilterTimeConstant=0.001  UdotUserProvided=0
  Simulink-PS Converter2 : nesl_utility/Simulink-PS Converter  PhysicalDomain=network_engine_domain  SubClassName=ps_input  LeftPortType=input  RightPortType=output  PseudoPeriodic=off  Frequencies=[]  NoiseDistribution=none  NoiseParameters=[]  Unit=degC  AffineConversion=on  FilteringAndDerivatives=provide  SimscapeFilterOrder=1  InputFilterTimeConstant=0.001  UdotUserProvided=0
  "Solver Configuration " : nesl_utility/Solver Configuration  PhysicalDomain=network_engine_domain  SubClassName=solver  LeftPortType=input  RightPortType=generic  Tones=[]  Harmonics=[]  SimulateNoise=off  Profile=off  UseLocalSampling=off  EnableSwitchedLinearOptims=on  FrequencyDomain=off  UseCCode=off  RelTol=0.001  AbsTol=0.001  MinStep=1e-09  ToWorkspace=off  RevertToSquareIcSolve=off  NumHomotopyIterations=100  PhasorMode=off  PhasorModeNumHarmonics=1  ConsistencySolver=NEWTON_XTOL_AFTER_FTOL  IndexReductionMethod=DerivativeReplacement  DoDC=off  ResidualTolerance=1e-09  ConsistencyTolSource=GLOBAL  ConsistencyAbsTol=0.001  ConsistencyRelTol=0.001  ConsistencyTolFactor=0.001  UseLocalSolver=off  LocalSolverChoice=NE_BACKWARD_EULER_ADVANCER  ResolveIndetEquations=on  FunctionEvalNumThread=1  LocalSolverSampleTime=0.001  DoFixedCost=off  MaxNonlinIter=3  MaxModeIter=2  ComputeImpulses=off  ImpulseIterations=2  LinearAlgebra=auto  LinearAlgebraNumThread=0  EquationFormulation=NE_TIME_EF  DelaysMemoryBudget=1024  AutomaticFiltering=on  FilteringTimeConstant=0.001  PartitionStorageMethod=AS_NEEDED  PartitionMemoryBudget=1024  PartitionMethod=ROBUST  MultibodyUseLocalSolver=off  MultibodyLocalSolverChoice=ODE1  MultibodyLocalSolverSampleTime=0.001
  T_4 : Outport
  wires:
  T_3/1 -> Simulink-PS Converter2/1
  T_a_4/1 -> Simulink-PS Converter1/1
  PS-Simulink Converter/1 -> T_4/1
  Q_4/1 -> Simulink-PS Converter/1
  connections:
  "Heater Heat Flow Source "/RConn2 -- " Thermal Reference"/LConn1 -- Neighbor 3 Temperature Source/RConn2 -- Ambient Temperature Source/RConn2 -- "Solver Configuration "/RConn1
  Room Thermal Mass/LConn1 -- Room Temperature Sensor/LConn1 -- "Heater Heat Flow Source "/LConn1 -- Ambient Thermal Resistance/RConn1 -- Neighbor 3 Thermal Resistance/RConn1
  Neighbor 3 Thermal Resistance/LConn1 -- Neighbor 3 Temperature Source/LConn1
  Room Temperature Sensor/RConn1 -- PS-Simulink Converter/LConn1
  Ambient Temperature Source/LConn1 -- Ambient Thermal Resistance/LConn1
  Neighbor 3 Temperature Source/RConn1 -- Simulink-PS Converter2/RConn1
  "Heater Heat Flow Source "/RConn1 -- Simulink-PS Converter/RConn1
  Simulink-PS Converter1/RConn1 -- Ambient Temperature Source/RConn1
